simulink model "RoadProfileGenerator"  (R2023a)
settings: Solver=VariableStepAuto  StartTime=0.0  StopTime=10.0  RelTol=1e-3
values from neighbouring files (symbols this model uses):
  v = 10    [Main.m]    (also in SweepTest.m; myActiveSuspensions.mat)
libraries: simulink x1
settings Model: Creator=aleze  LastModifiedBy=aleze

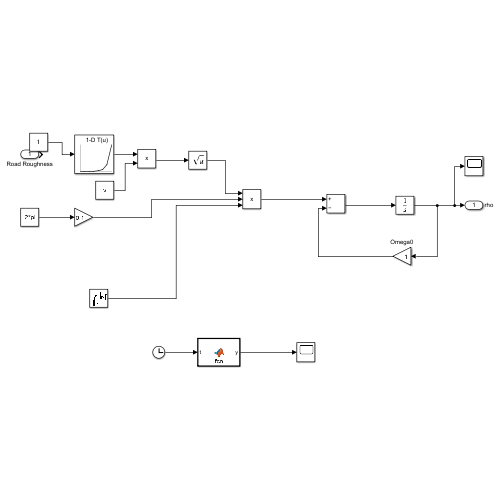
[thumbnail: Simulink's stored preview of the top-level diagram]
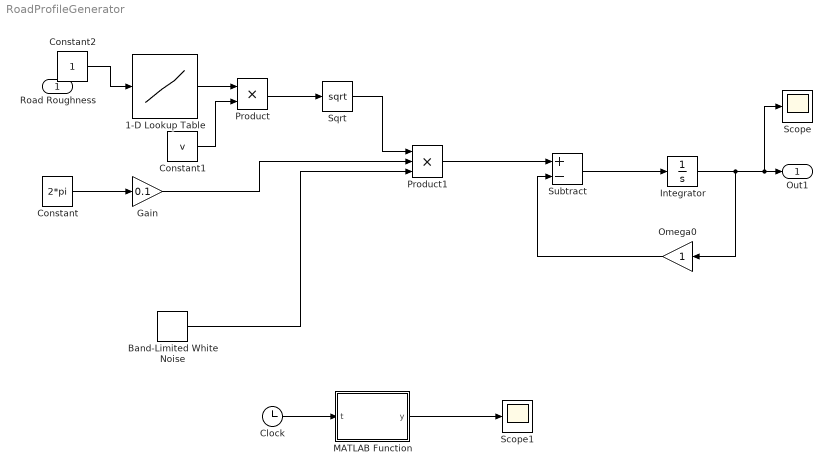
== system RoadProfileGenerator ==
  Road Roughness : Inport
  1-D Lookup Table : Lookup_n-D  NumberOfTableDimensions=1  BreakpointsForDimension1=[1;2;3;4;5;6;7;8]  Table=[1.6e-05;6.4e-05;0.000256;0.001024;0.004096;0.016384;0.065536;0.262144]  InternalRulePriority=Speed  RndMeth=Simplest
  Band-Limited White Noise : simulink/Sources/Band-Limited White Noise  Cov=0.001  Ts=0.01  seed=[23341]
  Clock : Clock
  Constant : Constant  Value=2*pi
  Constant1 : Constant  Value=v
  Constant2 : Constant
  Gain : Gain  Gain=0.1
  Integrator : Integrator
  MATLAB Function : MATLAB Function  TreatAsAtomicUnit=on
  Omega0 : Gain
  Product : Product
  Product1 : Product  Inputs=3
  Scope : Scope
  Scope1 : Scope
  Sqrt : Sqrt
  Subtract : Sum  Inputs=+-
  Out1 : Outport  SignalName=rho
  wires:
  Constant/1 -> Gain/1
  Constant1/1 -> Product/2
  1-D Lookup Table/1 -> Product/1
  Product/1 -> Sqrt/1
  Band-Limited White Noise/1 -> Product1/3
  Gain/1 -> Product1/2
  Sqrt/1 -> Product1/1
  Product1/1 -> Subtract/1
  Subtract/1 -> Integrator/1
  Integrator/1 -> Omega0/1, Scope/1, Out1/1
  Omega0/1 -> Subtract/2
  Constant2/1 -> 1-D Lookup Table/1
  Clock/1 -> MATLAB Function/1(t)
  MATLAB Function/1(y) -> Scope1/1

== matlab function RoadProfileGenerator/MATLAB Function ==
  data: t input; y output
function y = fcn(t)
r = 2;
if t<1
    y=0;
    
else
    if t>5
        y=0;
    else
   y = sqrt(r^2-(t-3)^2);
    end
end
